simulink model "xilinx_hw_test_au50_16k_8in"  (R2021a)
settings: Solver=VariableStepDiscrete  StartTime=0.0  StopTime=1024*2  RelTol=1e-3
undefined symbols (not defined in the file): d0, d1, d2, d3, d4, d5, d6, d7, sr
libraries: xbsIndex_r4 x1266, xrbsSSR_Library x13, casper_library_misc x7, xps_library x1
(part 5 of 18)

== system xilinx_hw_test_au50_16k_8in/bram_in6 ==
  addr : Inport
  data_in : Inport  Port=2
  we : Inport  Port=3
  Terminator : Terminator
  Terminator1 : Terminator
  Terminator2 : Terminator
  calc_add : Subsystem  mask{data_width=32, addr_width=11, sample_rate=sample_rate}
      mask prompts: data_width "data width"; addr_width "address width"; sample_rate "sample rate"
  convert_addr : xbsIndex_r4/Convert  gui_display_data_type=Fixed-point  arith_type=Unsigned  n_bits=addr_width  bin_pt=0  float_type=Single  exp_bits=8  fraction_bits=24  quantization=Truncate  overflow=Wrap  en=off  latency=0  pipeline=off  dbl_ovrd=off  block_type=convert
      settings: xl_area=[0, 0, 0, 0, 0, 0, 0]
  convert_din1 : xbsIndex_r4/Convert  gui_display_data_type=Fixed-point  arith_type=Unsigned  n_bits=32  bin_pt=0  float_type=Single  exp_bits=8  fraction_bits=24  quantization=Truncate  overflow=Wrap  en=off  latency=0  pipeline=off  dbl_ovrd=off  block_type=convert
      settings: xl_area=[0, 0, 0, 0, 0, 0, 0]
  convert_we : xbsIndex_r4/Convert  gui_display_data_type=Fixed-point  arith_type=Unsigned  n_bits=1  bin_pt=0  float_type=Single  exp_bits=8  fraction_bits=24  quantization=Truncate  overflow=Wrap  en=off  latency=0  pipeline=off  dbl_ovrd=off  block_type=convert
      settings: xl_area=[0, 0, 0, 0, 0, 0, 0]
  munge_in : Subsystem  AncestorBlock=casper_library_flow_control/munge  mask(munge){divisions=1, div_size=32, order=[0], arith_type_out=Unsigned, bin_pt_out=0}
      mask prompts: divisions "Number of divisions"; div_size "Division size (bits)"; order "Division packing order"; arith_type_out "Output arithmetic type"; bin_pt_out "Output binary point"
      mask help: Splits an input bus into the specified number of divisions and then recombines them in the order specified (most significant division = 0,least = number divisions-1)
      mask init:
      | munge_init(gcb, ...
      |     'divisions', divisions, ...
      |     'div_size', div_size, ...
      |     'order', order, ...
      |     'arith_type_out', arith_type_out, ...
      |     'bin_pt_out', bin_pt_out);
      settings: AttributesFormatString=|
      | split:32
      | join:0
      | Unsigned [32,0]
      mask TypeOptions arith_type_out: Unsigned | Signed  (2's comp) | Floating-point
  munge_out : Subsystem  AncestorBlock=casper_library_flow_control/munge  mask(munge){divisions=1, div_size=32, order=[0], arith_type_out=Signed  (2's comp), bin_pt_out=0}
      mask prompts: divisions "Number of divisions"; div_size "Division size (bits)"; order "Division packing order"; arith_type_out "Output arithmetic type"; bin_pt_out "Output binary point"
      mask help: Splits an input bus into the specified number of divisions and then recombines them in the order specified (most significant division = 0,least = number divisions-1)
      mask init:
      | munge_init(gcb, ...
      |     'divisions', divisions, ...
      |     'div_size', div_size, ...
      |     'order', order, ...
      |     'arith_type_out', arith_type_out, ...
      |     'bin_pt_out', bin_pt_out);
      settings: AttributesFormatString=|
      | split:32
      | join:0
      | Signed  (2's comp) [32,0]
      mask TypeOptions arith_type_out: Unsigned | Signed  (2's comp) | Floating-point
  sim_mem : Subsystem  mask{arith_type=Signed  (2's comp), addr_width=11, data_width=32, data_bin_pt=0, init_vals=[5793  -1458   4757   1335  -2579   6267  -4130   5928   5563  -7422   -739  -1014   1714   1726     95   -238   8345   3629  -1835   3599  -3355  -8095  10467  -2289   4898    711   1068  -3077   -699   1750  -4192   2955   6927  -1648    786   2632   -836   5736   1213  -3757   2783    579   6274  -6269   -321  -1127   8055   1612  -5108   5006   2466   1404   1625  -4794   3778  -9301   2006  -1493   1477  -1749   1774    942   2502  -6457  -6201     61  -5876   1668   1620   -902   4484 -13066    754  -5446   1608  -2616  -4606   4527   4601  -2884   9028  -3584   3461  -3652   2359   -738   9008  -4845  -3879   2315  -1416   2197   1295  -9118   4545   3868   9920 -10434   2524   1766  -7716   8394  -6696   2124   6728   2027  -2604  -1058    392   2434  -6210    -90   1863   2515  -4145   4722   -309  -1534   -410   -937   1026   5505  -3172  -1848    -34  -4085   1933   2778   3176  -3061   1535  -7446  10816  -3810   3442   4846   3576  -8299  -6720  -6133  -5295  -1533   -332  -6125   1895  -7377   -854 -13842  -2746  -1496  -3121  -4217   -418  -3629   6034  -5871   3414   1724  -2000   3516   6703    807    949   3303   7784   3579   5374   1128    611   2509  -2470   -276  -2156   7215     83  -1295   4694  -1272   2409   -354    -35  -1072   2062  -1304   2287  -7241   1632  -3711    749    -73  12007   -328  -6116  -4758   5796   2920  -5213  -1011     85  -3271   3603  -1153   3407  -5838   6625    894  -2563  -4260  -3703   3724  -5529  -2079   2216   -929   3073  -1164  -1039   7827  -3245  -4949   2454  -7344   2964  -8513   2321   1187   2078    120   3962  -2485  -1035     79  -3039 -11520   1544   1115   2083  -3776   1747  -2639   2572   6721  -5558   -629   -196  -3301   -435  -3604    987   4793    454  -1401  -4113  -3505   8573   -703   1067   4250   2288    843    844  -9882   3231  -4192   7850  -3413   5420    617   1423   2354    260  -2229   5491   4754  -1955  -4761   1357   2736  -4020   3685  -5469   -725   -591  -6913   4729  -8961  -1097  -1861  -1980  -4817   6878   4530   5829   1742   2099  -1039   1519    -88  -6150   4942   3072   -748   3452  -6451   1423   -298  -1334   5685   1108  -3301  -3889   6801   4618  -3570    704   7073   7454    908  -2455     60   5484   1720   -592   1964  -4191   5320   -436  -3537   3513   -579   1643   3247   1956  -5322  -7018   5587   2361   1940   4083   1090   7794    339    198   -122  -1713   2319   -269   3903   1339  -5275  -4283   -359   -612  -4921  -5226   5511   -594  -1202  -3264   3186   6632    887  -1350  -7498  -2838  -2942   8448  -8636   1780   -417    635    442   1932   2818   2656   1019  -3636  -7154  -8379  -2701  -4962   1748   4391  -1293  12207   -468  -5243    418   2027  -9762   -943   4844   5552  -2901   1181  -2547   1180   3153  -1358  -4467  -5583  -3660   6737   -705   2099  -9231  -2211  -5045   1068  -3313   5342  -3824   -604  -2695   5164   2568   2303    359   -632   1820   1168  -2211  -2903   1155   -617  -3766    923   -686   5281   -687   2666  -3916   5873  -4692   2895  -1330  -3480  -3864  -4268     53  -4036   3905    207   1848   6896  -3466   4289  -2050  -4070   2634   -257  -1749  -2708  -3577  -4121  -4180    124   3560   4934   5362     45     24    980  -2030  -5564   5123  -3506  -4698   8272   -807   1763  -6176     39    456   3717  -5041   8387   8001  -2779  -1673   6910   2581    470   7354   2616   2339  -2479  -2678   3572  -5958    -91   -373   7661   9428     34  -1784  -1330  -9353   4458  -6058   7233  -1631   1568   1943   -108  -7793   4948    444  -2576  -8878  -4062  -2435   3829  -4746   1969   1333  -1815   4873   1228  -4344   5974 -11327   -620  -7729   1518  -2284   3147  -4987   4488  -1954    -93   1445   1435   -247    655   6920  -1738  -1945   1459   4180    352   -656   3563  -9637  -5526   3468   6348  -4564  -2248   2286   7008   4791   5941  -6993   -193   1653    117   4227    805  -1302  -4477  -4543  -7900  -1264   1643   3959   -840  -7477   3328  -1944  -6758 ...(+10338 chars)], sample_rate=1, csp_latency=1}
      mask prompts: arith_type "Output Data Type"; addr_width "Address width"; data_width "Data width"; data_bin_pt "Data Binary Point"; init_vals "Initial values"; sample_rate "Sample rate"; csp_latency "Latency"
      mask init:
      | % set_param([gcb, '/data_to_xilinx'], 'arith_type', arith_type)
      | % set_param([gcb, '/data_to_xilinx'], 'n_bits', get_param(gcb, 'data_width'))
      mask TypeOptions arith_type: Unsigned | Signed  (2's comp)
      mask TypeOptions data_width: 8 | 16 | 32 | 64 | 128
  xilinx_hw_test_au50_16k_8in_bram_in6_addr : xbsIndex_r4/Gateway Out  inherit_from_input=off  hdl_port=on  rows=1  columns=1  UseAsDAC=off  DACChannel='1'  interface=None  automatic_assignment=on  address_offset=hex2dec('00')  intf_name=''  intf_description=''  timing_constraint=None  locs_specified=off  LOCs={'A5','B9','A9','C1','A3','G6','E9','A6','A7','A8','B8','B1','B3','D9','B5','B4','B6','C2'}  io_standard={}  block_type=gatewayout
      settings: infoedit="Gateway out block.  Converts Xilinx fixed point inputs into ouputs of type Simulink integer, double, or fixed point.<P><P>Hardware notes:  In hardware these blocks become top level output ports or are discarded, depending on how they are configured."  sginterface={'Nallatech'=>{'xdspkit'=>{'non_memory_mapped_port'=>'uprev_Shared_BRAM_addr'}},'Xilinx'=>{'jtaghwcosim'=>{'non_memory_mapped_port'=>'uprev_Shared_BRAM_addr'},'xdspkit'=>{'non_memory_mapped_port'=>'uprev_Shared_BRAM_addr'}}}  xl_area=[0, 0, 0, 0, 0, 0, 0]
  xilinx_hw_test_au50_16k_8in_bram_in6_data_in : xbsIndex_r4/Gateway Out  inherit_from_input=off  hdl_port=on  rows=1  columns=1  UseAsDAC=off  DACChannel='1'  interface=None  automatic_assignment=on  address_offset=hex2dec('00')  intf_name=''  intf_description=''  timing_constraint=None  locs_specified=off  LOCs={'B21','B22','A22','B23','B19','C19','A20','A21','A23','B24','A24','A25','E18','D18','C18','B18'}  io_standard={}  block_type=gatewayout
      settings: infoedit="Gateway out block.  Converts Xilinx fixed point inputs into ouputs of type Simulink integer, double, or fixed point.<P><P>Hardware notes:  In hardware these blocks become top level output ports or are discarded, depending on how they are configured."  sginterface={'Nallatech'=>{'xdspkit'=>{'non_memory_mapped_port'=>'uprev_Shared_BRAM_data_in'}},'Xilinx'=>{'jtaghwcosim'=>{'non_memory_mapped_port'=>'uprev_Shared_BRAM_data_in'},'xdspkit'=>{'non_memory_mapped_port'=>'uprev_Shared_BRAM_data_in'}}}  xl_area=[0, 0, 0, 0, 0, 0, 0]
  xilinx_hw_test_au50_16k_8in_bram_in6_data_out : xbsIndex_r4/Gateway In  gui_display_data_type=Fixed-point  arith_type=Unsigned  n_bits=32  bin_pt=0  preci_type=Single  exp_width=8  frac_width=24  rows=1  columns=1  quantization=Truncate  overflow=Wrap  period=sample_rate  UseAsADC=off  ADCChannel='1'  interface=None  automatic_assignment=on  address_offset=hex2dec('00')  intf_name=''  intf_description=''  default_value=0  timing_constraint=None  locs_specified=off  LOCs={}  io_standard={}  inherit_from_input=off  hdl_port=on  dbl_ovrd=off  block_type=gatewayin
      settings: xl_area=[0, 0, 0, 0, 0, 0, 0]
  xilinx_hw_test_au50_16k_8in_bram_in6_we : xbsIndex_r4/Gateway Out  inherit_from_input=off  hdl_port=on  rows=1  columns=1  UseAsDAC=off  DACChannel='1'  interface=None  automatic_assignment=on  address_offset=hex2dec('00')  intf_name=''  intf_description=''  timing_constraint=None  locs_specified=off  LOCs={'A14'}  io_standard={}  block_type=gatewayout
      settings: infoedit="Gateway out block.  Converts Xilinx fixed point inputs into ouputs of type Simulink integer, double, or fixed point.<P><P>Hardware notes:  In hardware these blocks become top level output ports or are discarded, depending on how they are configured."  xl_area=[0, 0, 0, 0, 0, 0, 0]
  data_out : Outport  VectorParamsAs1DForOutWhenUnconnected=off
  wires:
  munge_out/1(dout) -> data_out/1
  sim_mem/1(data_out) -> xilinx_hw_test_au50_16k_8in_bram_in6_data_out/1
  xilinx_hw_test_au50_16k_8in_bram_in6_data_out/1 -> munge_out/1(din)
  convert_addr/1 -> xilinx_hw_test_au50_16k_8in_bram_in6_addr/1
  convert_din1/1 -> xilinx_hw_test_au50_16k_8in_bram_in6_data_in/1
  data_in/1 -> munge_in/1(din)
  calc_add/1(out) -> convert_addr/1
  xilinx_hw_test_au50_16k_8in_bram_in6_we/1 -> Terminator2/1
  xilinx_hw_test_au50_16k_8in_bram_in6_data_in/1 -> Terminator1/1
  xilinx_hw_test_au50_16k_8in_bram_in6_addr/1 -> Terminator/1
  convert_we/1 -> xilinx_hw_test_au50_16k_8in_bram_in6_we/1
  addr/1 -> sim_mem/1(addr), calc_add/1(in)
  we/1 -> sim_mem/3(we), convert_we/1
  munge_in/1(dout) -> sim_mem/2(data), convert_din1/1

== system xilinx_hw_test_au50_16k_8in/bram_in7 ==
  addr : Inport
  data_in : Inport  Port=2
  we : Inport  Port=3
  Terminator : Terminator
  Terminator1 : Terminator
  Terminator2 : Terminator
  calc_add : Subsystem  mask{data_width=32, addr_width=11, sample_rate=sample_rate}
      mask prompts: data_width "data width"; addr_width "address width"; sample_rate "sample rate"
  convert_addr : xbsIndex_r4/Convert  gui_display_data_type=Fixed-point  arith_type=Unsigned  n_bits=addr_width  bin_pt=0  float_type=Single  exp_bits=8  fraction_bits=24  quantization=Truncate  overflow=Wrap  en=off  latency=0  pipeline=off  dbl_ovrd=off  block_type=convert
      settings: xl_area=[0, 0, 0, 0, 0, 0, 0]
  convert_din1 : xbsIndex_r4/Convert  gui_display_data_type=Fixed-point  arith_type=Unsigned  n_bits=32  bin_pt=0  float_type=Single  exp_bits=8  fraction_bits=24  quantization=Truncate  overflow=Wrap  en=off  latency=0  pipeline=off  dbl_ovrd=off  block_type=convert
      settings: xl_area=[0, 0, 0, 0, 0, 0, 0]
  convert_we : xbsIndex_r4/Convert  gui_display_data_type=Fixed-point  arith_type=Unsigned  n_bits=1  bin_pt=0  float_type=Single  exp_bits=8  fraction_bits=24  quantization=Truncate  overflow=Wrap  en=off  latency=0  pipeline=off  dbl_ovrd=off  block_type=convert
      settings: xl_area=[0, 0, 0, 0, 0, 0, 0]
  munge_in : Subsystem  AncestorBlock=casper_library_flow_control/munge  mask(munge){divisions=1, div_size=32, order=[0], arith_type_out=Unsigned, bin_pt_out=0}
      mask prompts: divisions "Number of divisions"; div_size "Division size (bits)"; order "Division packing order"; arith_type_out "Output arithmetic type"; bin_pt_out "Output binary point"
      mask help: Splits an input bus into the specified number of divisions and then recombines them in the order specified (most significant division = 0,least = number divisions-1)
      mask init:
      | munge_init(gcb, ...
      |     'divisions', divisions, ...
      |     'div_size', div_size, ...
      |     'order', order, ...
      |     'arith_type_out', arith_type_out, ...
      |     'bin_pt_out', bin_pt_out);
      settings: AttributesFormatString=|
      | split:32
      | join:0
      | Unsigned [32,0]
      mask TypeOptions arith_type_out: Unsigned | Signed  (2's comp) | Floating-point
  munge_out : Subsystem  AncestorBlock=casper_library_flow_control/munge  mask(munge){divisions=1, div_size=32, order=[0], arith_type_out=Signed  (2's comp), bin_pt_out=0}
      mask prompts: divisions "Number of divisions"; div_size "Division size (bits)"; order "Division packing order"; arith_type_out "Output arithmetic type"; bin_pt_out "Output binary point"
      mask help: Splits an input bus into the specified number of divisions and then recombines them in the order specified (most significant division = 0,least = number divisions-1)
      mask init:
      | munge_init(gcb, ...
      |     'divisions', divisions, ...
      |     'div_size', div_size, ...
      |     'order', order, ...
      |     'arith_type_out', arith_type_out, ...
      |     'bin_pt_out', bin_pt_out);
      settings: AttributesFormatString=|
      | split:32
      | join:0
      | Signed  (2's comp) [32,0]
      mask TypeOptions arith_type_out: Unsigned | Signed  (2's comp) | Floating-point
  sim_mem : Subsystem  mask{arith_type=Signed  (2's comp), addr_width=11, data_width=32, data_bin_pt=0, init_vals=[-2421   4171   2206  -4827   1367   2297  -2137   2927  -2954  -7174    905   1997  -3841  -3265   3587  -7786    232   1247    556  -3806  10149   4852   2955   -476   5662    -21  -5045   4604    771     40    322  -2100   -352  -4387  -1228  -1220    863    198  -4951   1237   5232   7107  -2435   -952  -3669   2995   9164  -1716  -3093  -2793    175  -1206   4245   1723   5882  -2450   -902   3664  -2977   2690  -2819   1084   9628   3322   1572    497   6250    -11   4728   1431   1744  -1482  -5280  -1218  -2719   3030   5098   3625   6964   4210  -8258   2237  -5280   4665   2337  -2781  -2357   8850   5417    774   3776   -351   3787   1513   -536  -8660   5393  -1050   -131  -4114   1534  -3585   4401  -8078  -4574   4966  -2716   5971   4520   4484  -3634  -2774  -9313    421   -264  -8002   -734    217    753  -4642   -837  -4884  -2411   4936   2883   -633    376   1631   3980   1443  -2891   -601   4323   -501   -384    634  -2606  -1099   4105   4054    497   4352  -3139   5384    558  -4447   1983   4400   2297   1473   5227  -2987  -1617  -6489   7481  -4489  -2959   1459   1429   1146   4891  -4476   -690    380   5316  -4774   2156  -4181   1674   2879   3569  -6544  -3503   3030   1867   7463  -4343  -1524    664  -6092   3939    499  -1874   1848   1391   2708   4712  -1891  -5460    847   3888  -7305   4445   -407    315   5599   -317  -2487  -3737  -2070   3040   3305   3862   4744   4160  -4826  -2059  -1430  -2439  -9037   2945  -9267   3373  -3081   -500  -8934  -2864   1172   2001  10914   6501  -3752  -4081   1572   2453    467   5924   1283  -1342   -686   1909   -259   7246  -6871  -1593   -750   3795    911    720  -5429   6027    813  -4523   2963   4193  -6675    530   -837   -531  -7538   5450   -667  -2980  -1589     79    944  -1188   2023  -2111  -1129   3923   5749    479   2568  -2288   1855   1832   1361   5173  -8558  -2237  -5095    718   1020  -1028  -6752  10132  -1457   5056   5474   1127  -6182   2599  -4276  -3994  -7547   6733  -1564   6177  -1678   5865   4531  -6184  -7844   -825   -952   1919  -3947   -109   2764  -2153   3736   4528    659  10421  -2066  -2025  -4545    932  -1162  -6442   2335   2045  -6753   3113   8036   8776   6747  -4581  -1748  -1418   -300   2105  -4601   1064   2123  -2320    763   -533  -2892   1435   2727   3041  -6338  -2822   1483   4664  -7580   2483  -3905   4359   1991  -1077   3941  -1501  -2702  -2797   7459   3275  -3414  -6872  -4092  -4004   1115   8885  -5311   4504   2703   1339  -2809   2348   3277   -585   5659   2987  -1883    507  -5089   5774   3728   1261  -3313   2674  -2949   -136    347   2398  -2607   6443   -864 -10255  -4249   5862   2217   2290   5454   5967  -2158   -590  -6073   3676  -1733  -4946  -2853   8833  -3941  -1620   -594   1643  -3301    938   2329  -2627   7691  -1614    927   1758  -6066    715   4828   2950   -922   2097  -1388  -3126  -3426   5468  -2153   2164  -2484   3315   5348   3359   -780   -814    206  -3296    220   -181  -3878   -614   4607   5074   4166   2505  -4931  -5439    867   -820   1903   5653  -4293   2350   1215  -3616  -3472   2937   4169   2302  -1031   2676    865   2619   2413   2339  -1993  -2173  -2423  -1364     -4  -7104  -7211  -2025   2023  -2057  -1227  -3934   5848   1196   5515   4163   -101   8115  -8027  -1681   3070   2168  -2488  -3120  -3592   2048   3454   1004   1909   1550  -2799  -1714   -657   1249  -4046   1628    787  -6970    465   4733  -4401   1562   3217  -3868  -8763  -6552   2792  -9724   -343   3121  -3568   4850   2206   3575   1405  -1153  -1731  -1525  -4564   1091 -10250   5992  -4644  -1396    886   1103   4381   1272   1347  -2360  -1665  10992   4234   2629 -12092     17    188   2491   2682  -3491  -3579  -4250   -305  -2574  -8214  -1466  -7308  -1324   2367   1400   1925   6556   -770   2070   3285   7375    535   1226  -6702  -1057   4706   1014  -6185   5460  -1051  -5215  -2509  -2125  -1145   4036   6700   3824   5452   3612  -1918  -3006 ...(+10337 chars)], sample_rate=1, csp_latency=1}
      mask prompts: arith_type "Output Data Type"; addr_width "Address width"; data_width "Data width"; data_bin_pt "Data Binary Point"; init_vals "Initial values"; sample_rate "Sample rate"; csp_latency "Latency"
      mask init:
      | % set_param([gcb, '/data_to_xilinx'], 'arith_type', arith_type)
      | % set_param([gcb, '/data_to_xilinx'], 'n_bits', get_param(gcb, 'data_width'))
      mask TypeOptions arith_type: Unsigned | Signed  (2's comp)
      mask TypeOptions data_width: 8 | 16 | 32 | 64 | 128
  xilinx_hw_test_au50_16k_8in_bram_in7_addr : xbsIndex_r4/Gateway Out  inherit_from_input=off  hdl_port=on  rows=1  columns=1  UseAsDAC=off  DACChannel='1'  interface=None  automatic_assignment=on  address_offset=hex2dec('00')  intf_name=''  intf_description=''  timing_constraint=None  locs_specified=off  LOCs={'A5','B9','A9','C1','A3','G6','E9','A6','A7','A8','B8','B1','B3','D9','B5','B4','B6','C2'}  io_standard={}  block_type=gatewayout
      settings: infoedit="Gateway out block.  Converts Xilinx fixed point inputs into ouputs of type Simulink integer, double, or fixed point.<P><P>Hardware notes:  In hardware these blocks become top level output ports or are discarded, depending on how they are configured."  sginterface={'Nallatech'=>{'xdspkit'=>{'non_memory_mapped_port'=>'uprev_Shared_BRAM_addr'}},'Xilinx'=>{'jtaghwcosim'=>{'non_memory_mapped_port'=>'uprev_Shared_BRAM_addr'},'xdspkit'=>{'non_memory_mapped_port'=>'uprev_Shared_BRAM_addr'}}}  xl_area=[0, 0, 0, 0, 0, 0, 0]
  xilinx_hw_test_au50_16k_8in_bram_in7_data_in : xbsIndex_r4/Gateway Out  inherit_from_input=off  hdl_port=on  rows=1  columns=1  UseAsDAC=off  DACChannel='1'  interface=None  automatic_assignment=on  address_offset=hex2dec('00')  intf_name=''  intf_description=''  timing_constraint=None  locs_specified=off  LOCs={'B21','B22','A22','B23','B19','C19','A20','A21','A23','B24','A24','A25','E18','D18','C18','B18'}  io_standard={}  block_type=gatewayout
      settings: infoedit="Gateway out block.  Converts Xilinx fixed point inputs into ouputs of type Simulink integer, double, or fixed point.<P><P>Hardware notes:  In hardware these blocks become top level output ports or are discarded, depending on how they are configured."  sginterface={'Nallatech'=>{'xdspkit'=>{'non_memory_mapped_port'=>'uprev_Shared_BRAM_data_in'}},'Xilinx'=>{'jtaghwcosim'=>{'non_memory_mapped_port'=>'uprev_Shared_BRAM_data_in'},'xdspkit'=>{'non_memory_mapped_port'=>'uprev_Shared_BRAM_data_in'}}}  xl_area=[0, 0, 0, 0, 0, 0, 0]
  xilinx_hw_test_au50_16k_8in_bram_in7_data_out : xbsIndex_r4/Gateway In  gui_display_data_type=Fixed-point  arith_type=Unsigned  n_bits=32  bin_pt=0  preci_type=Single  exp_width=8  frac_width=24  rows=1  columns=1  quantization=Truncate  overflow=Wrap  period=sample_rate  UseAsADC=off  ADCChannel='1'  interface=None  automatic_assignment=on  address_offset=hex2dec('00')  intf_name=''  intf_description=''  default_value=0  timing_constraint=None  locs_specified=off  LOCs={}  io_standard={}  inherit_from_input=off  hdl_port=on  dbl_ovrd=off  block_type=gatewayin
      settings: xl_area=[0, 0, 0, 0, 0, 0, 0]
  xilinx_hw_test_au50_16k_8in_bram_in7_we : xbsIndex_r4/Gateway Out  inherit_from_input=off  hdl_port=on  rows=1  columns=1  UseAsDAC=off  DACChannel='1'  interface=None  automatic_assignment=on  address_offset=hex2dec('00')  intf_name=''  intf_description=''  timing_constraint=None  locs_specified=off  LOCs={'A14'}  io_standard={}  block_type=gatewayout
      settings: infoedit="Gateway out block.  Converts Xilinx fixed point inputs into ouputs of type Simulink integer, double, or fixed point.<P><P>Hardware notes:  In hardware these blocks become top level output ports or are discarded, depending on how they are configured."  xl_area=[0, 0, 0, 0, 0, 0, 0]
  data_out : Outport  VectorParamsAs1DForOutWhenUnconnected=off
  wires:
  munge_out/1(dout) -> data_out/1
  sim_mem/1(data_out) -> xilinx_hw_test_au50_16k_8in_bram_in7_data_out/1
  xilinx_hw_test_au50_16k_8in_bram_in7_data_out/1 -> munge_out/1(din)
  convert_addr/1 -> xilinx_hw_test_au50_16k_8in_bram_in7_addr/1
  convert_din1/1 -> xilinx_hw_test_au50_16k_8in_bram_in7_data_in/1
  data_in/1 -> munge_in/1(din)
  calc_add/1(out) -> convert_addr/1
  xilinx_hw_test_au50_16k_8in_bram_in7_we/1 -> Terminator2/1
  xilinx_hw_test_au50_16k_8in_bram_in7_data_in/1 -> Terminator1/1
  xilinx_hw_test_au50_16k_8in_bram_in7_addr/1 -> Terminator/1
  convert_we/1 -> xilinx_hw_test_au50_16k_8in_bram_in7_we/1
  addr/1 -> sim_mem/1(addr), calc_add/1(in)
  we/1 -> sim_mem/3(we), convert_we/1
  munge_in/1(dout) -> sim_mem/2(data), convert_din1/1

== system xilinx_hw_test_au50_16k_8in/edge_detect ==
  in : Inport
  Delay : xbsIndex_r4/Delay  rst=off  infoeditControl=Selection of Reset will increase slice count due to use of real FFs and instead of SRLs  en=off  latency=1  reg_retiming=off  dbl_ovrd=off  block_type=delay
      settings: xl_area=[0, 0, 0, 0, 0, 0, 0]
  Inverter : xbsIndex_r4/Inverter  en=off  latency=0  dbl_ovrd=off  block_type=inv
      settings: xl_area=[0, 0, 0, 0, 0, 0, 0]
  edge_op : xbsIndex_r4/Logical  logical_function=NOR  inputs=2  en=off  latency=0  precision=Full  arith_type=Unsigned  n_bits=8  bin_pt=2  align_bp=on  dbl_ovrd=off  block_type=logical
      settings: xl_area=[0, 0, 0, 0, 0, 0, 0]
  out : Outport  VectorParamsAs1DForOutWhenUnconnected=off
  wires:
  Inverter/1 -> edge_op/1
  edge_op/1 -> out/1
  in/1 -> Inverter/1, Delay/1
  Delay/1 -> edge_op/2

== system xilinx_hw_test_au50_16k_8in/edge_detect1 ==
  in : Inport
  Delay : xbsIndex_r4/Delay  rst=off  infoeditControl=Selection of Reset will increase slice count due to use of real FFs and instead of SRLs  en=off  latency=1  reg_retiming=off  dbl_ovrd=off  block_type=delay
      settings: xl_area=[0, 0, 0, 0, 0, 0, 0]
  Inverter : xbsIndex_r4/Inverter  en=off  latency=0  dbl_ovrd=off  block_type=inv
      settings: xl_area=[0, 0, 0, 0, 0, 0, 0]
  edge_op : xbsIndex_r4/Logical  logical_function=NOR  inputs=2  en=off  latency=0  precision=Full  arith_type=Unsigned  n_bits=8  bin_pt=2  align_bp=on  dbl_ovrd=off  block_type=logical
      settings: xl_area=[0, 0, 0, 0, 0, 0, 0]
  out : Outport  VectorParamsAs1DForOutWhenUnconnected=off
  wires:
  Inverter/1 -> edge_op/1
  edge_op/1 -> out/1
  in/1 -> Inverter/1, Delay/1
  Delay/1 -> edge_op/2

== system xilinx_hw_test_au50_16k_8in/in_enable ==
  sim_1 : Inport
  convert1_1 : DataTypeConversion  OutDataTypeStr=fixdt('ufix1_En0')  LockScale=on
  convert2_1 : DataTypeConversion  OutDataTypeStr=fixdt('ufix1_En0')  ConvertRealWorld=Stored Integer (SI)  LockScale=on
  gain_1 : Gain  OutDataTypeStr=fixdt('ufix32_En0')
  io_delay : xbsIndex_r4/Delay  rst=off  infoeditControl=Selection of Reset will increase slice count due to use of real FFs and instead of SRLs  en=off  latency=0  reg_retiming=on  dbl_ovrd=off  block_type=delay
  slice_reg : xbsIndex_r4/Slice  nbits=1  boolean_output=on  mode=Lower Bit Location + Width  bit1=0  base1=MSB of Input  bit0=0  base0=LSB of Input  dbl_ovrd=off  block_type=slice
  xilinx_hw_test_au50_16k_8in_in_enable_user_data_out : xbsIndex_r4/Gateway In  gui_display_data_type=Fixed-point  arith_type=Unsigned  n_bits=32  bin_pt=0  preci_type=Single  exp_width=8  frac_width=24  rows=1  columns=1  quantization="Round  (unbiased: +/- Inf)"  overflow=Saturate  period=1  UseAsADC=off  ADCChannel='1'  interface=None  automatic_assignment=on  address_offset=hex2dec('00')  intf_name=''  intf_description=''  default_value=0  timing_constraint=None  locs_specified=off  LOCs={}  io_standard={}  inherit_from_input=off  hdl_port=on  dbl_ovrd=off  block_type=gatewayin
  in_reg : Outport  VectorParamsAs1DForOutWhenUnconnected=off
  wires:
  xilinx_hw_test_au50_16k_8in_in_enable_user_data_out/1 -> io_delay/1
  sim_1/1 -> convert1_1/1
  convert1_1/1 -> convert2_1/1
  convert2_1/1 -> gain_1/1
  gain_1/1 -> xilinx_hw_test_au50_16k_8in_in_enable_user_data_out/1
  io_delay/1 -> slice_reg/1
  slice_reg/1 -> in_reg/1
